simulink model "WingSim"  (Simulink 7.4)
settings: Solver=ode45  StartTime=0  StopTime=1  FixedStep=ts  RelTol=1e-3
model workspace (MAT data in the model file):
  ts : num (value not decoded)
values from neighbouring files (symbols this model uses):
  simRunner = SimRunner('simRunner')    [testSimRunner.m]
libraries: mblibv1 x2, cstblocks x1, FlutterLib x1, simulink x1
settings Model: Creator=Rafal  ModifiedByFormat=Rafal  LastModifiedBy=Rafal  ExtModeArmWhenConnect=off  BufferReuse=off
settings Model: ModifiedComment=|
  | Rafal -- Sat Feb 23 17:53:04 2013 -- Version 1.346
  | Turbulence applied directly to alpha calculation (not U0)
settings Model: ModifiedHistory=|
  | Rafal -- Sat Feb 23 17:53:04 2013 -- Version 1.346
  | Turbulence applied directly to alpha calculation (not U0)
  | 
  | Rafal -- Sat Feb 23 17:44:49 2013 -- Version 1.345
  | Fix turbulence
  | 
  | Rafal -- Sat Feb 23 17:32:06 2013 -- Version 1.344
  | Turbulence. Only w is used (not w_dot)
  | 
  | Rafal -- Sat Feb 23 17:22:58 2013 -- Version 1.343
  | Turbulence added
  | 
  | Rafal -- Thu Feb 07 20:03:51 2013 -- Version 1.342
  | 
  | 
  | Rafal -- Thu Feb 07 20:02:41 2013 -- Version 1.341
  | 
  | 
  | Rafal -- Thu Feb 07 20:01:15 2013 -- Version 1.340
  | 
  | 
  | Rafal -- Thu Feb 07 19:10:07 2013 -- Version 1.339
  | Mask Wing subystem
  | 
  | Rafal -- Thu Feb 07 19:00:08 2013 -- Version 1.338
  | Wing subsystem moved to shared library
  | 
  | Rafal -- Thu Feb 07 18:59:31 2013 -- Version 1.337
  | Wing subsystem removed to shared library
  | 
  | Rafal -- Tue Feb 05 00:13:44 2013 -- Version 1.336
  | 
  | 
  | Rafal -- Tue Feb 05 00:12:22 2013 -- Version 1.335
  | 
  | 
  | Rafal -- Mon Feb 04 19:51:08 2013 -- Version 1.334
  | 
  | 
  | Rafal -- Mon Feb 04 19:14:36 2013 -- Version 1.333
  | 
  | 
  | Rafal -- Mon Feb 04 19:09:34 2013 -- Version 1.332
  | 
  | 
  | Rafal -- Mon Feb 04 19:01:45 2013 -- Version 1.331
  | 
  | 
  | Rafal -- Mon Feb 04 18:55:54 2013 -- Version 1.330
  | 
  | 
  | Rafal -- Mon Feb 04 18:24:17 2013 -- Version 1.329
  | 
  | 
  | Rafal -- Mon Feb 04 18:17:49 2013 -- Version 1.328
  | 
  | 
  | Rafal -- Mon Feb 04 02:04:22 2013 -- Version 1.327
  | 
  | 
  | Rafal -- Mon Feb 04 02:00:31 2013 -- Version 1.326
  | 
  | 
  | Rafal -- Mon Feb 04 01:01:05 2013 -- Version 1.325
  | 
  | 
  | Rafal -- Mon Feb 04 00:56:31 2013 -- Version 1.324
  | 
  | 
  | Rafal -- Mon Feb 04 00:48:55 2013 -- Version 1.323
  | SimRunner
  | 
  | Rafal -- Sun Feb 03 22:29:11 2013 -- Version 1.322
  | 
  | 
  | Rafal -- Sun Feb 03 22:11:10 2013 -- Version 1.321
  | 
  | 
  | Rafal -- Sun Feb 03 22:09:23 2013 -- Version 1.320
  | No initFcn
  | 
  | Rafal -- Fri Feb 01 00:20:34 2013 -- Version 1.319
  | 
  | 
  | Rafal -- Thu Jan 31 23:56:09 2013 -- Version 1.318
  | 
  | 
  | Rafal -- Thu Jan 31 23:45:26 2013 -- Version 1.317
  | 
  | 
  | Rafal -- Thu Jan 31 23:37:18 2013 -- Version 1.316
  | 
  | 
  | Rafal -- Thu Jan 31 23:32:50 2013 -- Version 1.315
  | 
  | 
  | Rafal -- Thu Jan 31 23:31:24 2013 -- Version 1.314
  | 
  | 
  | Rafal -- Sun Jan 20 23:13:45 2013 -- Version 1.313
  | Korzystamy z zewnetrznych parametrow bactParams, dumpBact
  | Dla danych z BACT wyniki pokrywaja sie idealnie z modelem analitycznym i modelem z Matlab files exchange
  | 
  | Rafal -- Sun Jan 20 20:08:58 2013 -- Version 1.312
  | 
  | 
  | Rafal -- Sun Jan 20 20:07:59 2013 -- Version 1.311
  | 
  | 
  | Rafal -- Sun Jan 20 20:04:53 2013 -- Version 1.310
  | 
  | 
  | Rafal -- Sun Jan 20 19:07:50 2013 -- Version 1.309
  | 
  | 
  | Rafal -- Sun Jan 20 18:53:01 2013 -- Version 1.308
  | 
  | 
  | Rafal -- Fri Jan 18 13:35:31 2013 -- Version 1.307
  | 
  | 
  | Rafal -- Thu Jan 17 00:20:40 2013 -- Version 1.306
  | 
  | 
  | Rafal -- Wed Jan 16 23:53:54 2013 -- Version 1.305
  | 
  | 
  | Rafal -- Wed Jan 16 23:42:52 2013 -- Version 1.304
  | Dodana konfiguracjaL CriticalSpeed do oszacowania predkosci krytycznej.
  | 
  | Rafal -- Wed Jan 16 19:50:35 2013 -- Version 1.303
  | Fix na linearyzacje.
  | Wczesniej Alpha_dot =  Alpha -> du/dt
  | Teraz:
  | Wywalony bloczek 'du/dt'.
  | Alpha_dot = Theta_dot - H_dot_dot/U0
  | Pochodna h_dot_dot wzieta bezposrednio z bloczku Wing Body
  | 
  | Rafal -- Wed Jan 16 15:02:06 2013 -- Version 1.302
  | 
  | 
  | Rafal -- Wed Jan 16 11:27:09 2013 -- Version 1.301
  | Turbulence addedd
settings DataIOCC: InitialState=simState  LimitDataPoints=off  LoadExternalInput=on  SaveState=on  SignalLogging=off  SignalLoggingName=sigsOut
settings OptimizationCC: BlockReduction=off  InlineParams=on  OptimizeBlockIOStorage=off  BufferReuse=off  EnforceIntegerDowncast=off  ExpressionFolding=off  FoldNonRolledExpr=off  LocalBlockOutputs=off  InitFltsAndDblsToZero=on
settings DebuggingCC: AlgebraicLoopMsg=none  SaveWithParameterizedLinksMsg=none  SignalResolutionControl=TryResolveAllWithWarning  SolverPrmCheckMsg=none  MultiTaskDSMMsg=warning  MultiTaskCondExecSysMsg=none  UnconnectedInputMsg=none  UnconnectedOutputMsg=none  UnconnectedLineMsg=none  StrictBusMsg=None
settings HardwareCC: TargetUnknown=on
settings RTWCC: SystemTargetFile=xpctarget.tlc  TemplateMakefile=xpc_default_tmf  ProcessScript=xpctarget_make_rtw_hook  IncludeERTFirstTime=on
settings TargetCC: TargetFcnLib=ansi_tfl_tmw.mat  TargetFunctionLibrary=ANSI_C  IsPILTarget=off  CompOptLevelCompliant=off  MatFileLogging=on  EnableShiftOperators=on  PortableWordSizes=off
settings CustomProperty: DataType=string  Value=Real-Time
settings SimscapeCC: SelectedTab=SimMechanics

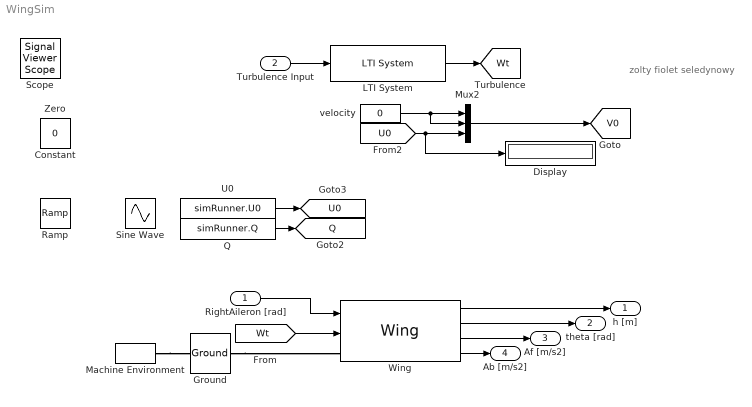
== system WingSim ==
  note: zolty
      | fiolet
      | seledynowy
  RightAileron [rad] : Inport  OutDataType=fixdt(1, 16)  OutScaling=2^0
  Turbulence Input : Inport  Port=2  OutDataType=fixdt(1, 16)  OutScaling=2^0
  Display : Display
  Ground : mblibv1/Bodies/Ground  DialogController=MECH.DynMechDlgSource  SystemSampleTime=-1  UpdateFromCAD=off  LeftPortType=env  RightPortType=workingframe  PhysicalDomain=Mechanical  DialogClass=GroundBlock  CoordPosition=[0 0 0]  CoordPositionUnits=m  StateVectorMgrId=19  MachineId=[20 0]  ShowEnvPort=on
  LTI System : cstblocks/LTI System  SystemSampleTime=-1  sys=simRunner.turbulence  IC=[]
  Machine Environment : mblibv1/Bodies/Machine Environment  DialogController=MECH.DialogSource  SystemSampleTime=-1  PortType=env  PhysicalDomain=Mechanical  DialogTemplateClass=MECH.MachineEnvironment  SyncWhenCopied=off  Gravity=[0 -simRunner.g 0]  GravityUnits=m/s^2  GravityAsSignal=off  Dimensionality=3D Only  AnalysisType=Forward dynamics  LinearAssemblyTolerance=1e-3  LinearAssemblyToleranceUnits=m  AngularAssemblyTolerance=1e-3  AngularAssemblyToleranceUnits=rad  ConstraintSolverType=Stabilizing  ConstraintRelTolerance=1e-4  ConstraintAbsTolerance=1e-4  UseRobustSingularityHandling=off  RedundancyAnalysisToleranceType=Automatically select tolerance  RedundancyAnalysisTolerance=1e-14  StatePerturbationType=Adaptive  PerturbationSize=1e-3  VisualizeMachine=on  BodyVisualizationType=Use model default body geometries  BodyColorSelMode=Use model default  DefaultBodyColor=[1 0 0]
  Mux2 : Mux  Inputs=3
  Q : Constant  Value=simRunner.Q  OutDataType=sfix(16)  OutScaling=2^0
  U0 : Constant  Value=simRunner.U0  OutDataType=sfix(16)  OutScaling=2^0
  Wing : FlutterLib/Wing  SystemSampleTime=-1  wing=simRunner.wingParams  wingOrientation=[0 0 0]
  velocity : Constant  Value=0  OutDataType=sfix(16)  OutScaling=2^0
  h [m] : Outport  OutDataType=fixdt(1, 16)  OutScaling=2^0
  theta [rad] : Outport  Port=2  OutDataType=fixdt(1, 16)  OutScaling=2^0
  Af [m/s2] : Outport  Port=3  OutDataType=fixdt(1, 16)  OutScaling=2^0
  Ab [m/s2] : Outport  Port=4  OutDataType=fixdt(1, 16)  OutScaling=2^0
  Constant : Constant  IOType=siggen  Value=-1  OutDataType=sfix(16)  OutScaling=2^0
  Ramp : simulink/Sources/Ramp  IOType=siggen  SystemSampleTime=-1  slope=1  start=0  X0=0
  Scope : SignalViewerScope  IOType=viewer  ZoomMode=xonly  LegendLocations="674.3333      275.3333            95            41"  RefreshTime=0.035000
      settings: ShowLegends=on  YMin=-0.0018  YMax=0.0002
  Sine Wave : Sin  IOType=siggen  Amplitude=10  Bias=0  Frequency=5  Phase=pi/2  Samples=10  SampleTime=0  Offset=0
  Zero : Constant  IOType=siggen  Value=0  OutDataType=sfix(16)  OutScaling=2^0
  tag scope: Q=global, U0=global, V0=global, Wt=global
  wires:
  [U0] -> Mux2/3, Display/1
  Wing/2 -> theta [rad]/1
  Mux2/1 -> [V0]
  U0/1 -> [U0]
  Q/1 -> [Q]
  RightAileron [rad]/1 -> Wing/1
  Wing/1 -> h [m]/1
  Wing/3 -> Af [m/s2]/1
  Wing/4 -> Ab [m/s2]/1
  Turbulence Input/1 -> LTI System/1
  velocity/1 -> Mux2/1, Mux2/2
  LTI System/1 -> [Wt]
  [Wt] -> Wing/2
  connections:
  Machine Environment/RConn1 -- Ground/LConn1
  Ground/RConn1 -- Wing/LConn1
